simulink model "Boost_and_bidirectionalconv_latest"  (R2022b)
settings: Solver=ode45  StartTime=0.0  StopTime=10  RelTol=1e-3
undefined symbols (not defined in the file): Ion, Lithium
libraries: spsMosfetLib x7, spsSeriesRLCBranchLib x6, spsCurrentMeasurementLib x2, spsMeanLib x2, spsPWMGeneratorDCDCLib x2, spsVoltageMeasurementLib x2, spsDiodeLib x1, spsACVoltageSourceLib x1, simulink x1, spsBistableLib x1, spsBatteryLib x1, slpidlib x1
settings Model: Creator=LENOVO  LastModifiedBy=LENOVO
settings DataIOCC: ReturnWorkspaceOutputs=off
settings DebuggingCC: AlgebraicLoopMsg=none  UnconnectedInputMsg=warning  UnconnectedOutputMsg=warning  UnconnectedLineMsg=warning  SFMachineParentedDataDiag=warning  ArithmeticOperatorsInVariantConditions=warning
settings ModelReferenceCC: EnableRefExpFcnMdlSchedulingChecks=on
settings SFSimCC: CustomCodeUndefinedFunction=UseInterfaceOnly

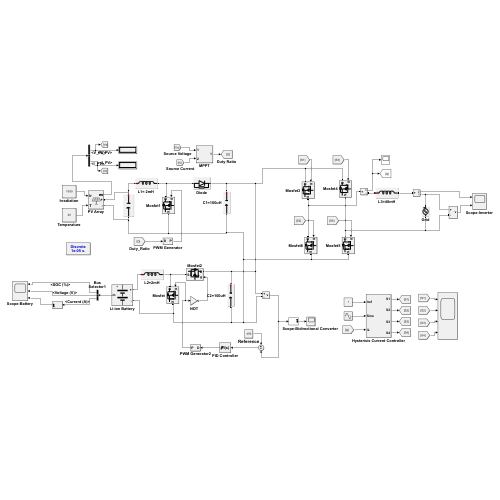
[thumbnail: Simulink's stored preview of the top-level diagram]
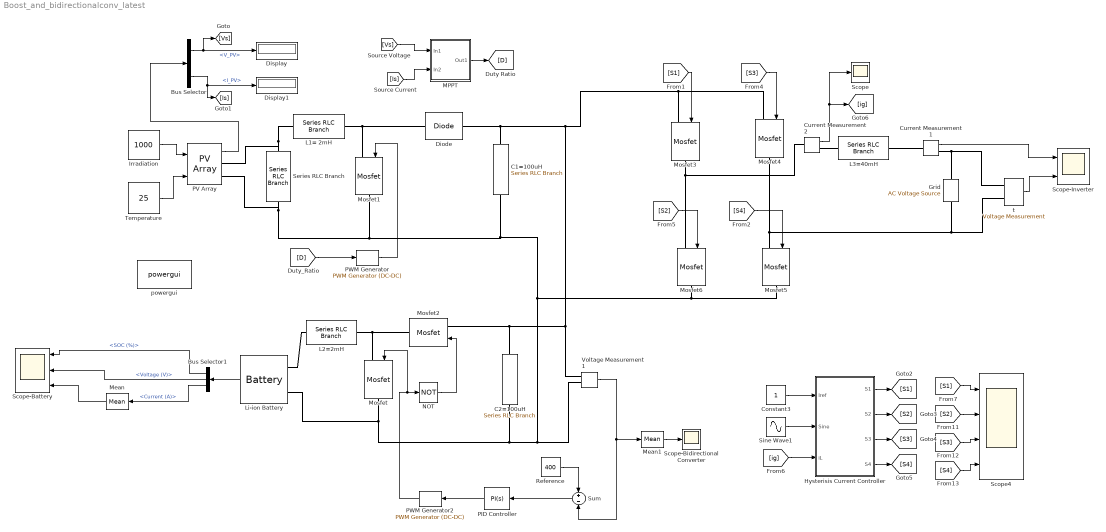
== system Boost_and_bidirectionalconv_latest ==
  Bus Selector : BusSelector  OutputSignals=V_PV,I_PV
  Bus Selector1 : BusSelector  OutputSignals=SOC (%),Voltage (V),Current (A)
  C1=100uH : spsSeriesRLCBranchLib/Series RLC Branch  LConnTagsString=__new0  RConnTagsString=__new0  BranchType=C  Resistance=1  Inductance=1e-3  SetiL0=off  InitialCurrent=0  Capacitance=100e-6  Setx0=off  InitialVoltage=0  Measurements=None
  C2=100uH : spsSeriesRLCBranchLib/Series RLC Branch  LConnTagsString=__new0  RConnTagsString=__new0  BranchType=C  Resistance=1  Inductance=1e-3  SetiL0=off  InitialCurrent=0  Capacitance=100e-6  Setx0=off  InitialVoltage=0  Measurements=None
  Constant3 : Constant
  Current Measurement1 : spsCurrentMeasurementLib/Current Measurement  PhasorSimulation=off  OutputType=Complex  PSBequivalent=0
  Current Measurement2 : spsCurrentMeasurementLib/Current Measurement  PhasorSimulation=off  OutputType=Complex  PSBequivalent=0
  Diode : spsDiodeLib/Diode  Ron=0.001  Lon=0  Vf=0.8  IC=0  UseSnubber=0  Rs=500  Cs=250e-9  Measurements=off
  Display : Display
  Display1 : Display
  Grid : spsACVoltageSourceLib/AC Voltage Source  Amplitude=325  Phase=0  Frequency=50  SampleTime=0  Measurements=None  BusType=swing  Pref=10e3  Qref=0  Qmin=-inf  Qmax=+inf
  Hysterisis Current Controller : Subsystem
  Irradiation : Constant  Value=1000
  "L1= 2mH " : spsSeriesRLCBranchLib/Series RLC Branch  LConnTagsString=__new0  RConnTagsString=__new0  BranchType=L  Resistance=1  Inductance=2e-3  SetiL0=off  InitialCurrent=0  Capacitance=1e-6  Setx0=off  InitialVoltage=0  Measurements=None
  L2=2mH : spsSeriesRLCBranchLib/Series RLC Branch  LConnTagsString=__new0  RConnTagsString=__new0  BranchType=L  Resistance=1  Inductance=2e-3  SetiL0=off  InitialCurrent=0  Capacitance=1e-6  Setx0=off  InitialVoltage=0  Measurements=None
  L3=40mH : spsSeriesRLCBranchLib/Series RLC Branch  LConnTagsString=__new0  RConnTagsString=__new0  BranchType=L  Resistance=1  Inductance=40e-3  SetiL0=off  InitialCurrent=0  Capacitance=1e-6  Setx0=off  InitialVoltage=0  Measurements=None
  Li-ion Battery : spsBatteryLib/Battery  BatType=Lithium-Ion  ShowTempParam=off  ThermalPreset=no  ShowAgeParam=off  NomV=100  NomQ=20  SOC=60  Batt_Tr=30  PresetModel=on  MaxQ=20  MinV=75  FullV=116.3987  Dis_rate=8.6957  R=0.05  Normal_OP=18.087  expZone="[108.0386     0.9826087]"  current=[6.5 13 32.5]  Units=Time  Tci=20  NomT=20  T2=-30  MaxQ2=4.8  FullV2=7.1  Normal_OP2=5.655  expZone2="[6.58           1]"  Rca=0.6  ti=2000  Dp=0  Neq0=0  Tsim=1e6  Ta1=25  Qeol=5.4*0.9  Reol=0.013333*1.2  Char_age=[2.3478, 3]  Dis_age=[2.3478, 10]  N1=1500  N2=10500  N3=1000  N4=1400  Ta2=45  N5=950
  MPPT : Subsystem
  Mean : spsMeanLib/Mean  Freq=50  Vinit=0  Ts=0
  Mean1 : spsMeanLib/Mean  Freq=60  Vinit=0  Ts=0
  Mosfet : spsMosfetLib/Mosfet  Ron=0.001  Lon=0  Rd=0.01  Vfd=0  IC=0  Rs=1e5  Cs=inf  Measurements=off
  Mosfet1 : spsMosfetLib/Mosfet  Ron=0.001  Lon=0  Rd=0.01  Vfd=0  IC=0  Rs=1e5  Cs=inf  Measurements=off
  Mosfet2 : spsMosfetLib/Mosfet  Ron=0.001  Lon=0  Rd=0.01  Vfd=0  IC=0  Rs=1e5  Cs=inf  Measurements=off
  Mosfet{3..6} (4 alike) : spsMosfetLib/Mosfet  Ron=0.1  Lon=0  Rd=0.01  Vfd=0  IC=0  Rs=1e5  Cs=inf  Measurements=off
  "NOT " : Logic  Operator=NOT  IconShape=distinctive  AllPortsSameDT=off  OutDataTypeStr=boolean
  PID Controller : slpidlib/PID Controller  Controller=PI  Form=Parallel  TimeDomain=Continuous-time  UseExternalTs=off  SampleTime=-1  IntegratorMethod=Forward Euler  FilterMethod=Forward Euler  ControllerParametersSource=internal  P=0.0002  I=0.01  UseKiTs=off  D=0  N=100  UseFilter=on  TunerSelectOption=Transfer Function Based (PID Tuner App)  InitialConditionSource=internal  InitialConditionForIntegrator=0  InitialConditionForFilter=0  DifferentiatorICPrevScaledInput=0  ExternalReset=none  TrackingMode=off  Kt=1  LimitOutput=on  SatLimitsSource=internal  UpperSaturationLimit=0.9  LowerSaturationLimit=0  LinearizeAsGain=on  AntiWindupMode=none  Kb=1  LimitIntegrator=off  UpperIntegratorSaturationLimit=inf  LowerIntegratorSaturationLimit=-inf  POutMin=[]  POutMax=[]  IOutMin=[]  IOutMax=[]  DOutMin=[]  DOutMax=[]  NOutMin=[]  NOutMax=[]  SumOutMin=[]  SumOutMax=[]  SaturationOutMin=[]  SaturationOutMax=[]  PParamMin=[]  PParamMax=[]  IParamMin=[]  IParamMax=[]  DParamMin=[]  DParamMax=[]  NParamMin=[]  NParamMax=[]  KbParamMin=[]  KbParamMax=[]  KtParamMin=[]  KtParamMax=[]  KbOutMin=[]  KbOutMax=[]  KtOutMin=[]  KtOutMax=[]  IntegratorOutMin=[]  IntegratorOutMax=[]  FilterOutMin=[]  FilterOutMax=[]  SumI1OutMin=[]  SumI1OutMax=[]  SumI2OutMin=[]  SumI2OutMax=[]  SumI3OutMin=[]  SumI3OutMax=[]  SumI4OutMin=[]  SumI4OutMax=[]  SumDOutMin=[]  SumDOutMax=[]  DifferentiatorOutMin=[]  DifferentiatorOutMax=[]  FilterDiffOutCoefMin=[]  FilterDiffOutCoefMax=[]  ReciprocalOutMin=[]  ReciprocalOutMax=[]  SumDenOutMin=[]  SumDenOutMax=[]  SumNumOutMin=[]  SumNumOutMax=[]  DivideOutMin=[]  DivideOutMax=[]  UdiffTsProdOutMin=[]  UdiffTsProdOutMax=[]  NTsProdOutMin=[]  NTsProdOutMax=[]  UintegralTsProdOutMin=[]  UintegralTsProdOutMax=[]  UngainTsProdOutMin=[]  UngainTsProdOutMax=[]  ClampingZeroOutDataTypeStr=Inherit: Inherit via back propagation  ClampingZeroOutMin=[]  ClampingZeroOutMax=[]  FilterDenConstantOutDataTypeStr=Inherit: Inherit via back propagation  FilterDenConstantOutMin=[]  FilterDenConstantOutMax=[]  PCopyOutDataTypeStr=Inherit: Inherit via back propagation  PCopyOutMin=[]  PCopyOutMax=[]  NCopyOutDataTypeStr=Inherit: Inherit via back propagation  NCopyOutMin=[]  NCopyOutMax=[]  IntegratorContinuousStateAttributes=''  IntegratorStateMustResolveToSignalObject=off  IntegratorRTWStateStorageClass=Auto  FilterContinuousStateAttributes=''  FilterStateMustResolveToSignalObject=off  FilterRTWStateStorageClass=Auto  ParallelPVariant=InternalParameters  IdealPVariant=Disabled  IVariant=InternalParameters  DVariant=Disabled  IntegratorVariant=Continuous  SatVariant=Enabled  AWVariant=Passthrough  PCopyVariant=Disabled  TRVariant=Disabled  FdbkBlocksVariant=Forward  IdealPFdbkVariant=Disabled  SatFdbkVariant=Disabled  DerivativeFilterVariant=Disabled  NVariant=Disabled  NCopyVariant=Disabled_SignalSpec  FilterICVariant=Disabled  IntegratorICVariant=InternalICs  ExternalResetVariant=Disabled  TRSumVariant=Passthrough  SumFdbkVariant=Disabled  SumVariant=Sum_PI  TsampFilterVariant=InternalTs  TsampNgainVariant=Passthrough  TsampIntegralVariant=Passthrough  ExternalSaturationOutDataTypeStr=Inherit: Same as second input
  PV Array : spsPVArrayLib/PV Array  Npar=1  Nser=5  PlotType=array @ 1000 W/m2 & specified temperatures  S_vec="[ 1000  500  100 ]"  Temp_C_vec="[ 45 25  ]"  ModuleName=Global Solar Energy FG-2BTM-100  PlotWhenSelected=off  Pm=99.68  Ncell=36  Voc=23.3  Isc=6.4  Vm=17.8  Im=5.6  beta_Voc_pc=-0.326  alpha_Isc_pc=0.006  beta_Voc=-0.075958  alpha_Isc=0.000384  IL=6.4895  I0=5.5956e-11  nI=0.99289  Rsh=36.0927  Rs=0.50476  RobustModel=off  RobustCellTemperature=313.3991  BAL=off  Tc=1e-6  Tfilter=5e-5
  "PWM Generator " : spsPWMGeneratorDCDCLib/PWM Generator (DC-DC)  Fsw=30000  Ts=0
  PWM Generator2 : spsPWMGeneratorDCDCLib/PWM Generator (DC-DC)  Fsw=30000  Ts=0
  Reference : Constant  Value=400
  Scope : Scope
  Scope-Battery : Scope  NumInputPorts=3
  "Scope-Bidirectional Converter " : Scope
  Scope-Inverter : Scope  NumInputPorts=2
  Scope4 : Scope  NumInputPorts=4
  Series RLC Branch : spsSeriesRLCBranchLib/Series RLC Branch  LConnTagsString=__new0  RConnTagsString=__new0  BranchType=C  Resistance=1  Inductance=1e-3  SetiL0=off  InitialCurrent=0  Capacitance=100e-6  Setx0=off  InitialVoltage=0  Measurements=None
  Sine Wave1 : Sin  Frequency=2*pi*50  SampleTime=0
  Sum : Sum  Inputs=+-
  Temperature : Constant  Value=25
  Voltage Measurement1 : spsVoltageMeasurementLib/Voltage Measurement  PhasorSimulation=off  OutputType=Complex  PSBequivalent=0
  powergui : spspowerguiLib/powergui  Priority=1  SimulationMode=Discrete  SampleTime=10e-06  frequency=60  Iterations=50  frequencyindice=0  Pbase=100e6  ErrMax=1e-4  UnitsV=kV  UnitsW=MW  buscounter=0  FunctionMessages=off  echomessages=off  EnableUseOfTLC=off  CurrentSourceSwitches=off  DisableSnubberDevices=off  DisableRonSwitches=off  DisableVfSwitches=off  DisplayEquations=off  AutomaticDiscreteSolvers=off  SolverType=Tustin/Backward Euler (TBE)  Interpol=off  ExternalGateDelay=off  methode=off  Ts=100  x0status=blocks  SPID=off  SwTol=0  HookPort=off  NonlinearTolerance=1e-4  nMaxIteration=100  ContinueOnMaxIteration=off  RestoreLinks=warning  ResistiveCurrentMeasurement=off  Frange=[0:2:500]  Ylog=off  Xlog=on  ShowGrid=off  save=off  variable=ZData  structure=0  ZoomFFT=off  StartTime=0.0  cycles=1  DisplayStyle=1  fundamental=60  FreqAxis=off  MaxFrequency=1000  frequencyindicesteady=1  RmsSteady=1  display=off
  t : spsVoltageMeasurementLib/Voltage Measurement  PhasorSimulation=off  OutputType=Complex  PSBequivalent=0
  wires:
  Temperature/1 -> PV Array/2
  Irradiation/1 -> PV Array/1
  PV Array/1 -> Bus Selector/1
  Bus Selector/1 -> Display/1, [Vs]  "<V_PV>"
  Bus Selector/2 -> [Is], Display1/1  "<I_PV>"
  [D] -> "PWM Generator "/1
  "PWM Generator "/1 -> Mosfet1/1
  [Vs] -> MPPT/1(In1)
  [Is] -> MPPT/2(In2)
  MPPT/1(Out1) -> [D]
  "NOT "/1 -> Mosfet2/1
  Sum/1 -> PID Controller/1
  PID Controller/1 -> PWM Generator2/1
  Reference/1 -> Sum/1
  PWM Generator2/1 -> "NOT "/1, Mosfet/1
  Voltage Measurement1/1 -> Mean1/1, Sum/2
  Li-ion Battery/1 -> Bus Selector1/1
  Bus Selector1/1 -> Scope-Battery/1  "<SOC (%)>"
  Bus Selector1/2 -> Scope-Battery/2  "<Voltage (V)>"
  Bus Selector1/3 -> Mean/1  "<Current (A)>"
  Mean/1 -> Scope-Battery/3
  [S1] -> Mosfet3/1
  t/1 -> Scope-Inverter/2
  Hysterisis Current Controller/4(S4) -> [S4]
  Sine Wave1/1 -> Hysterisis Current Controller/2(Sine)
  [ig] -> Hysterisis Current Controller/3(iL)
  Constant3/1 -> Hysterisis Current Controller/1(Iref)
  [S3] -> Mosfet4/1
  Hysterisis Current Controller/2(S2) -> [S2]
  [S4] -> Mosfet5/1
  Hysterisis Current Controller/3(S3) -> [S3]
  [S2] -> Mosfet6/1
  Hysterisis Current Controller/1(S1) -> [S1]
  [S3] -> Scope4/3
  [S2] -> Scope4/2
  [S4] -> Scope4/4
  [S1] -> Scope4/1
  Current Measurement1/1 -> Scope-Inverter/1
  Mean1/1 -> "Scope-Bidirectional Converter "/1
  Current Measurement2/1 -> [ig], Scope/1
  connections:
  PV Array/RConn1 -- "L1= 2mH "/LConn1 -- Series RLC Branch/LConn1
  Series RLC Branch/RConn1 -- PV Array/RConn2 -- Mosfet1/RConn1 -- Voltage Measurement1/LConn2 -- Mosfet/RConn1 -- Li-ion Battery/LConn2 -- C2=100uH/RConn1 -- Mosfet6/RConn1 -- Mosfet5/RConn1 -- C1=100uH/RConn1
  Diode/LConn1 -- Mosfet1/LConn1 -- "L1= 2mH "/RConn1
  L2=2mH/RConn1 -- Mosfet/LConn1 -- Mosfet2/RConn1
  Li-ion Battery/LConn1 -- L2=2mH/LConn1
  Mosfet5/LConn1 -- Grid/LConn1 -- t/LConn2 -- Mosfet4/RConn1
  t/LConn1 -- Grid/RConn1 -- Current Measurement1/RConn1
  Current Measurement1/LConn1 -- L3=40mH/RConn1
  Mosfet6/LConn1 -- Current Measurement2/LConn1 -- Mosfet3/RConn1
  Diode/RConn1 -- C1=100uH/LConn1 -- Mosfet3/LConn1 -- Mosfet4/LConn1 -- Voltage Measurement1/LConn1 -- Mosfet2/LConn1 -- C2=100uH/LConn1
  Current Measurement2/RConn1 -- L3=40mH/LConn1

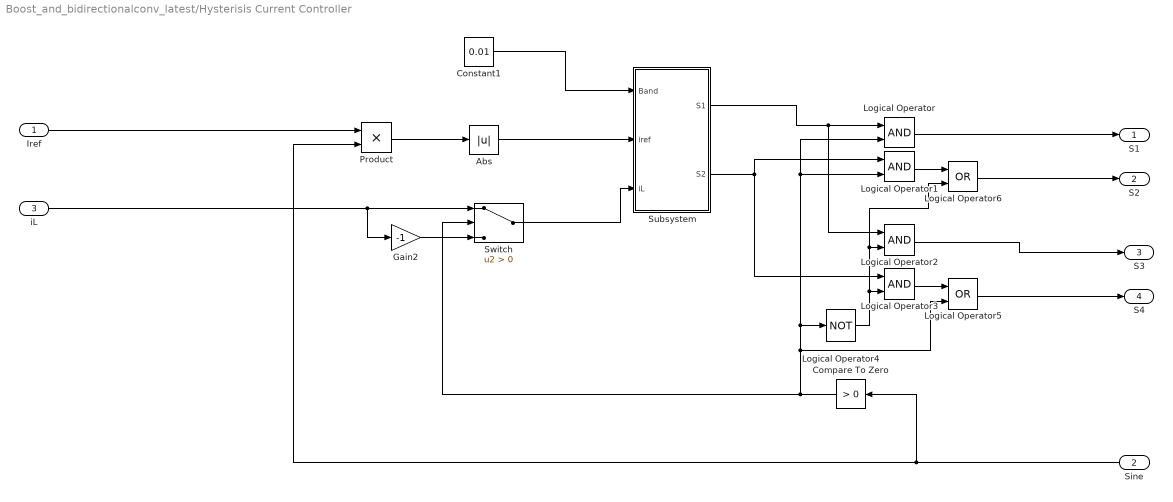
== system Boost_and_bidirectionalconv_latest/Hysterisis Current Controller ==
  Iref : Inport
  Sine : Inport  Port=2
  iL : Inport  Port=3
  Abs : Abs  SaturateOnIntegerOverflow=off
  Compare To Zero : simulink/Logic and Bit Operations/Compare To Zero  relop=>  OutDataTypeStr=boolean
  Constant1 : Constant  Value=0.01
  Gain2 : Gain  Gain=-1
  Logical Operator{,1..3} (4 alike) : Logic  AllPortsSameDT=off  OutDataTypeStr=boolean
  Logical Operator4 : Logic  Operator=NOT  AllPortsSameDT=off  OutDataTypeStr=boolean
  Logical Operator5 : Logic  Operator=OR  AllPortsSameDT=off  OutDataTypeStr=boolean
  Logical Operator6 : Logic  Operator=OR  AllPortsSameDT=off  OutDataTypeStr=boolean
  Product : Product
  Subsystem : Subsystem
  Switch : Switch  Criteria=u2 > Threshold  SaturateOnIntegerOverflow=off  InputSameDT=off
  S1 : Outport  VectorParamsAs1DForOutWhenUnconnected=off
  S2 : Outport  Port=2  VectorParamsAs1DForOutWhenUnconnected=off
  S3 : Outport  Port=3  VectorParamsAs1DForOutWhenUnconnected=off
  S4 : Outport  Port=4  VectorParamsAs1DForOutWhenUnconnected=off
  wires:
  Subsystem/2(S2) -> Logical Operator3/1, Logical Operator1/1
  Subsystem/1(S1) -> Logical Operator/1, Logical Operator2/1
  Constant1/1 -> Subsystem/1(Band)
  Product/1 -> Abs/1
  Switch/1 -> Subsystem/3(iL)
  Abs/1 -> Subsystem/2(iref)
  Compare To Zero/1 -> Logical Operator5/2, Logical Operator/2, Logical Operator1/2, Logical Operator4/1, Switch/2
  Logical Operator3/1 -> Logical Operator5/1
  Logical Operator2/1 -> S3/1
  Gain2/1 -> Switch/3
  Sine/1 -> Compare To Zero/1, Product/2
  Logical Operator4/1 -> Logical Operator3/2, Logical Operator2/2, Logical Operator6/2
  Iref/1 -> Product/1
  Logical Operator/1 -> S1/1
  iL/1 -> Gain2/1, Switch/1
  Logical Operator6/1 -> S2/1
  Logical Operator5/1 -> S4/1
  Logical Operator1/1 -> Logical Operator6/1

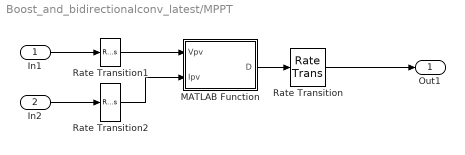
== system Boost_and_bidirectionalconv_latest/MPPT ==
  In1 : Inport
  In2 : Inport  Port=2
  MATLAB Function : MATLAB Function  TreatAsAtomicUnit=on
  Rate Transition : RateTransition  OutPortSampleTime=1e-7
  Rate Transition1 : RateTransition  OutPortSampleTime=1e-3
  Rate Transition2 : RateTransition  OutPortSampleTime=1e-3
  Out1 : Outport
  wires:
  In1/1 -> Rate Transition1/1
  MATLAB Function/1(D) -> Rate Transition/1
  Rate Transition2/1 -> MATLAB Function/2(Ipv)
  Rate Transition1/1 -> MATLAB Function/1(Vpv)
  Rate Transition/1 -> Out1/1
  In2/1 -> Rate Transition2/1

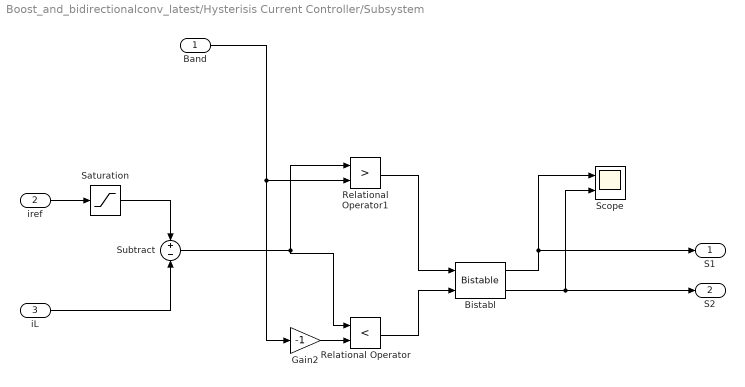
== system Boost_and_bidirectionalconv_latest/Hysterisis Current Controller/Subsystem ==
  Band : Inport
  iref : Inport  Port=2
  iL : Inport  Port=3
  Bistabl : spsBistableLib/Bistable  Qpriority=Set  ic=0  Ts=0
  Gain2 : Gain  Gain=-1
  Relational Operator : RelationalOperator  Operator=<  OutDataTypeStr=boolean  RndMeth=Simplest  InputSameDT=off
  Relational Operator1 : RelationalOperator  Operator=>  OutDataTypeStr=boolean  RndMeth=Simplest  InputSameDT=off
  Saturation : Saturate  UpperLimit=10  LowerLimit=0
  Scope : Scope  NumInputPorts=2
  Subtract : Sum  Inputs=+-
  S1 : Outport  VectorParamsAs1DForOutWhenUnconnected=off
  S2 : Outport  Port=2  VectorParamsAs1DForOutWhenUnconnected=off
  wires:
  Gain2/1 -> Relational Operator/2
  Band/1 -> Gain2/1, Relational Operator1/2
  Subtract/1 -> Relational Operator/1, Relational Operator1/1
  Bistabl/1 -> S1/1, Scope/1
  Bistabl/2 -> S2/1, Scope/2
  iL/1 -> Subtract/2
  Saturation/1 -> Subtract/1
  Relational Operator/1 -> Bistabl/2
  iref/1 -> Saturation/1
  Relational Operator1/1 -> Bistabl/1

== matlab function Boost_and_bidirectionalconv_latest/MPPT/MATLAB Function ==
  data: Vpv input; D output; Ipv input
function D = atom(Vpv,Ipv)
   persistent Dprev Vprev Pprev 
 
  if isempty(Dprev)
   Dprev = 0.5;
   Pprev= 76.5;
   Vprev = 20.5;

  end
detla_d = 0.001;
Ppv = Vpv*Ipv;
   if (Ppv-Pprev)~=0
       
       if (Ppv-Pprev) >0
           
          if (Vpv-Vprev)>0
              D = Dprev-detla_d;
          else
              D = Dprev+detla_d;
          end
          
       else
           
           if (Vpv-Vprev)>0
              D= Dprev+detla_d;
          else
              D = Dprev-detla_d;
           end
       end
   else
       D = Dprev;

   end 
   Dprev = D;
   Vprev = Vpv;
   Pprev = Ppv;
